simulink model "PX4OutputMappingHex"  (R2024a)
settings: configuration reference "standardSILConfiguraitonParams" (kept outside this file)
undefined symbols (not defined in the file): MotorCommandHexBus
settings Model: Creator=jerem  LastModifiedBy=jerem
settings ConfigSetRef: SourceName=standardSILConfiguraitonParams  SourceLocation=Base Workspace

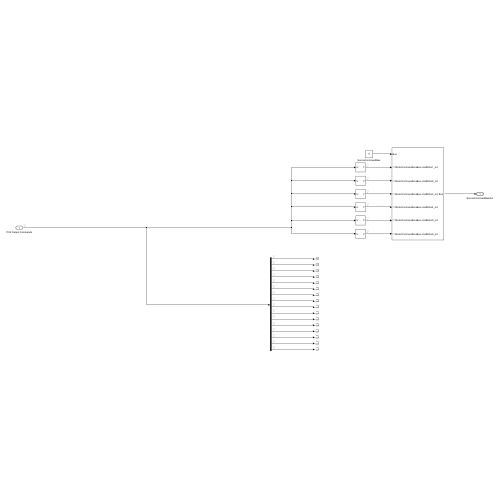
[thumbnail: Simulink's stored preview of the top-level diagram]
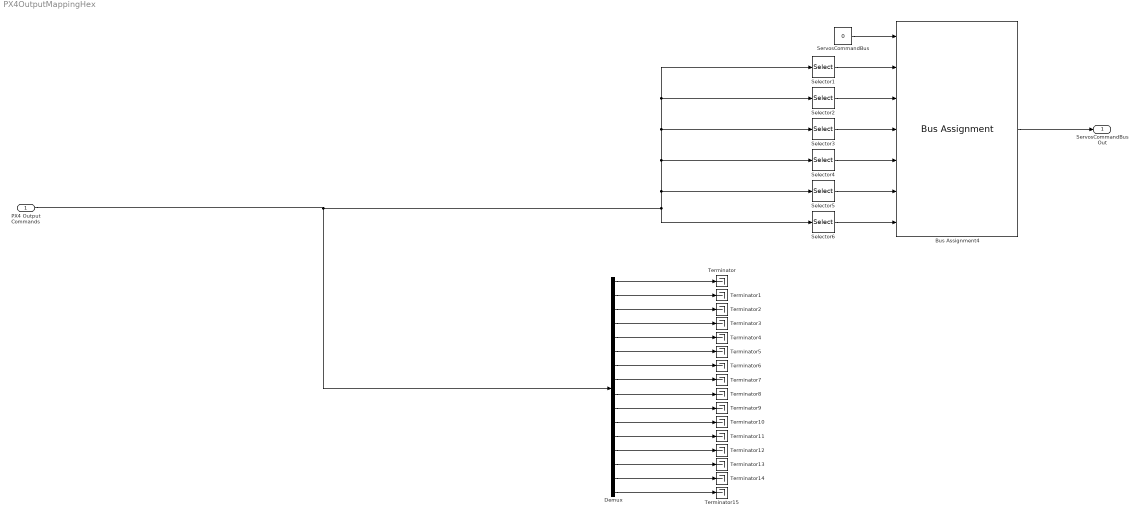
== system PX4OutputMappingHex ==
  PX4 Output Commands : Inport  PortDimensions=16
  Bus Assignment4 : BusAssignment  AssignedSignals=MotorCommandHexBus.cmdRotor1_nd,MotorCommandHexBus.cmdRotor2_nd,MotorCommandHexBus.cmdRotor3_nd,MotorCommandHexBus.cmdRotor4_nd,MotorCommandHexBus.cmdRotor5_nd,MotorCommandHexBus.cmdRotor6_nd
  Demux : Demux  Outputs=16
  Selector1 : Selector  InputPortWidth=16  IndexOptions=Index vector (dialog)  Indices=1  OutputSizes=1
  Selector2 : Selector  InputPortWidth=16  IndexOptions=Index vector (dialog)  Indices=2  OutputSizes=1
  Selector3 : Selector  InputPortWidth=16  IndexOptions=Index vector (dialog)  Indices=3  OutputSizes=1
  Selector4 : Selector  InputPortWidth=16  IndexOptions=Index vector (dialog)  Indices=4  OutputSizes=1
  Selector5 : Selector  InputPortWidth=16  IndexOptions=Index vector (dialog)  Indices=5  OutputSizes=1
  Selector6 : Selector  InputPortWidth=16  IndexOptions=Index vector (dialog)  Indices=6  OutputSizes=1
  ServosCommandBus : Constant  Value=0  OutDataTypeStr=Bus: ServosCommandBus
  Terminator{,1..15} (16 alike) : Terminator
  ServosCommandBusOut : Outport  OutDataTypeStr=Bus: ServosCommandBus
  wires:
  ServosCommandBus/1 -> Bus Assignment4/1
  Bus Assignment4/1 -> ServosCommandBusOut/1
  PX4 Output Commands/1 -> Demux/1, Selector1/1, Selector2/1, Selector3/1, Selector4/1, Selector5/1, Selector6/1
  Demux/1 -> Terminator/1
  Demux/2 -> Terminator1/1
  Demux/4 -> Terminator3/1
  Demux/3 -> Terminator2/1
  Demux/5 -> Terminator4/1
  Demux/6 -> Terminator5/1
  Demux/7 -> Terminator6/1
  Demux/8 -> Terminator7/1
  Demux/9 -> Terminator8/1
  Demux/10 -> Terminator9/1
  Demux/11 -> Terminator10/1
  Demux/12 -> Terminator11/1
  Demux/13 -> Terminator12/1
  Demux/14 -> Terminator13/1
  Demux/15 -> Terminator14/1
  Demux/16 -> Terminator15/1
  Selector1/1 -> Bus Assignment4/2
  Selector2/1 -> Bus Assignment4/3
  Selector3/1 -> Bus Assignment4/4
  Selector4/1 -> Bus Assignment4/5
  Selector5/1 -> Bus Assignment4/6
  Selector6/1 -> Bus Assignment4/7
